simulink model "EngPrt_TrqLimCalc"  (R2018a)
settings: configuration reference "cs_ert" (kept outside this file)
settings Model: DataDictionary=EngPrt_TrqLimCalc.sldd  Creator=zhoutinglin  LastModifiedBy=zhoutinglin

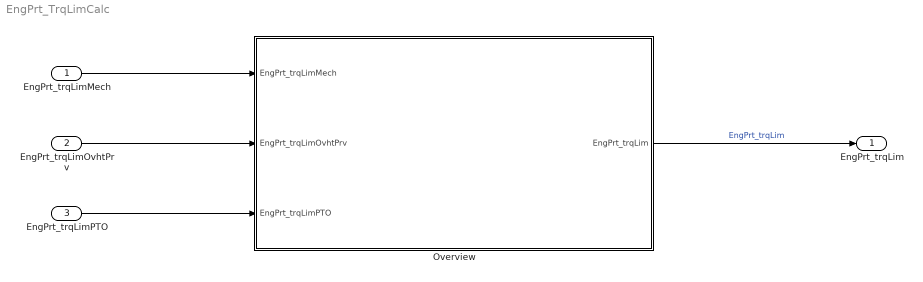
== system EngPrt_TrqLimCalc ==
  EngPrt_trqLimMech : Inport  Description=Resulting limiting torque for engine mechanics protection (inner engine torque)  OutMin=-3276.8  OutMax=3276.7  OutDataTypeStr=Torq  Unit=Nm  PortDimensions=[1 1]
  EngPrt_trqLimOvhtPrv : Inport  Description=Torque limitation value for engine protection from overheating  Port=2  OutMin=-3276.8  OutMax=3276.7  OutDataTypeStr=Torq  Unit=Nm  PortDimensions=[1 1]
  EngPrt_trqLimPTO : Inport  Description=Torque limitation value from PTO state  Port=3  OutMin=-3276.8  OutMax=3276.7  OutDataTypeStr=Torq  Unit=Nm  PortDimensions=[1 1]
  Overview : Subsystem
  EngPrt_trqLim : Outport
  wires:
  EngPrt_trqLimMech/1 -> Overview/1(EngPrt_trqLimMech)
  EngPrt_trqLimOvhtPrv/1 -> Overview/2(EngPrt_trqLimOvhtPrv)
  EngPrt_trqLimPTO/1 -> Overview/3(EngPrt_trqLimPTO)
  Overview/1(EngPrt_trqLim) -> EngPrt_trqLim/1  "EngPrt_trqLim"

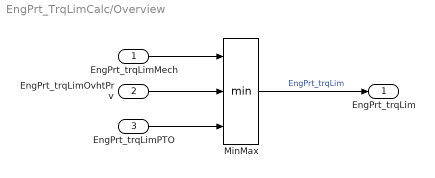
== system EngPrt_TrqLimCalc/Overview ==
  EngPrt_trqLimMech : Inport  Tag=Nm
  EngPrt_trqLimOvhtPrv : Inport  Tag=Nm  Port=2
  EngPrt_trqLimPTO : Inport  Tag=Nm  Port=3
  MinMax : MinMax  Inputs=3
  EngPrt_trqLim : Outport  Tag=Nm
  wires:
  EngPrt_trqLimOvhtPrv/1 -> MinMax/2
  EngPrt_trqLimPTO/1 -> MinMax/3
  MinMax/1 -> EngPrt_trqLim/1  "EngPrt_trqLim"
  EngPrt_trqLimMech/1 -> MinMax/1
